simulink model "variant_subsys"  (R2021b)
settings: Solver=VariableStepAuto  StartTime=0.0  StopTime=10.0  RelTol=1e-3
settings Model: Creator=fredric  LastModifiedBy=fredric

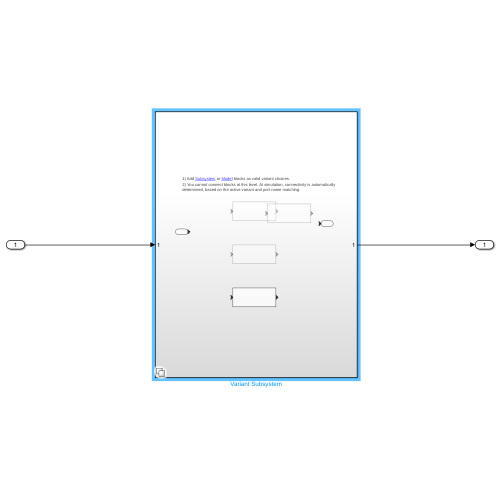
[thumbnail: Simulink's stored preview of the top-level diagram]
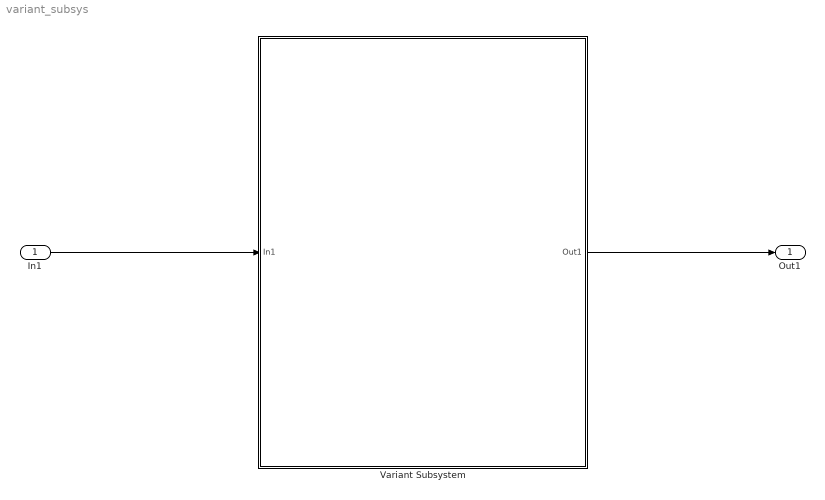
== system variant_subsys ==
  In1 : Inport
  Variant Subsystem : Subsystem  Variant=on
  Out1 : Outport
  wires:
  In1/1 -> Variant Subsystem/1(In1)
  Variant Subsystem/1(Out1) -> Out1/1

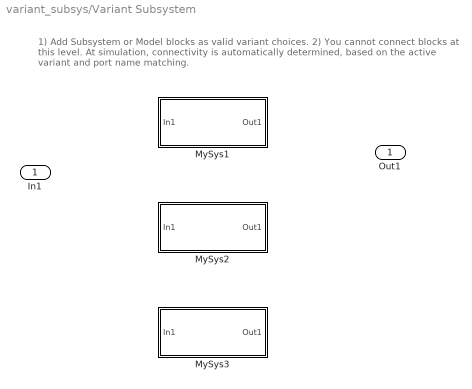
== system variant_subsys/Variant Subsystem ==
  note: 1) Add Subsystem or Model blocks as valid variant choices.
      | 2) You cannot connect blocks at this level. At simulation, connectivity is automatically
      | determined, based on the active variant and port name matching.
  In1 : Inport
  MySys1 : Subsystem  VariantControl=KK == 1
  MySys2 : Subsystem  VariantControl=KK == 2
  MySys3 : Subsystem  VariantControl=KK == 3
  Out1 : Outport

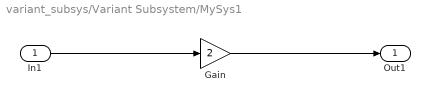
== system variant_subsys/Variant Subsystem/MySys1 ==
  In1 : Inport
  Gain : Gain  Gain=2
  Out1 : Outport
  wires:
  In1/1 -> Gain/1
  Gain/1 -> Out1/1

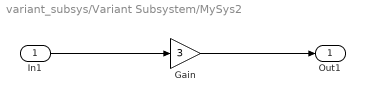
== system variant_subsys/Variant Subsystem/MySys2 ==
  In1 : Inport
  Gain : Gain  Gain=3
  Out1 : Outport
  wires:
  In1/1 -> Gain/1
  Gain/1 -> Out1/1

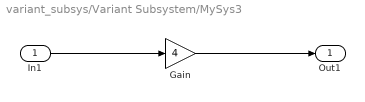
== system variant_subsys/Variant Subsystem/MySys3 ==
  In1 : Inport
  Gain : Gain  Gain=4
  Out1 : Outport
  wires:
  In1/1 -> Gain/1
  Gain/1 -> Out1/1
